simulink model "AllPurposeModel_TyreRelaxation"  (R2013b)
settings: Solver=ode45  StartTime=0.0  StopTime=16  FixedStep=0.001  MaxStep=0.01  RelTol=1e-3
StopFcn:
  | PlotPathAndForces(pos_irp3,delta_w4,F_z4,v_xv4,v_yv4,F_xv4,F_yv4, Par, -2);
  | TimePlots
undefined symbols (not defined in the file or in its folder): Par, sigbuilder_block
(part 1 of 2)
settings Model: DSRTSU_INTERNAL_RTI_VER=440  DSRTSU_INTERNAL_RTI_TYPE=rti1401  RTICANMMDATA=struct('GeneralSetupData',struct('modelroot','D:\Users\bengtja\Subversion_work\TM_VEAS_VD\CourseMaterial\MMF062_VehicleDynamics\Compendium\AllPurposeModel','generalsettings',struct('filesettings',struct('destfolder',struct('Name','RTICANMM_FILES','Check',1),'buildfolder',struct('Name','.','Check',1),'AbsDestfolder',struct('Name','D:\Users\bengtja\Subversion_work\TM_VEAS_VD\CourseMaterial\MMF062_VehicleDynamics\Compendium\AllPurposeModel\RTICANMM_FILES'),'AbsBuildfolder',struct('Name','D:\Users\bengtja\Subversion_work\TM_VEAS_VD\CourseMaterial\MMF062_VehicleDynamics\Compendium\AllPurposeModel'))),'options',struct('addpaths',1,'rmpaths',1,'addtrcexclusion',logical(1),'cannavigator',struct('checkmonitoring',0),'show_usrtrc',0,'use_usrtrc',0),'advanced',struct('options',[1 1 1 1 1 1 1 1 1 1 1 1 1 1 1 1 1 1 1 1 1 1 1 1 1 1 1 1 1 1 1 1 1 1 1 1 1 1 1 1 1 1 1 1 1 1 1 1 1 1 1 1 1 1 1 1 1 1 1 1 1 1 1 1 1 1 1 1 1 1 1 1 1 1 1 1 1 1 1 1 1 1 1 1 1 1 1 1 1 1 1 1 1 1 1 1 1 1 1 1]),'MPSetup',{{}},'modelname','AllPurposeModel','block','AllPurposeModel'))  DSRTSU_INTERNAL_RTIFPGA=30  BufferReuse=off  Creator=bengtja  LastModifiedBy=bengtja
settings OptimizationCC: BlockReduction=off  OptimizeBlockIOStorage=off  BufferReuse=off  ExpressionFolding=off  LocalBlockOutputs=off
settings DebuggingCC: ArtificialAlgebraicLoopMsg=none  StateNameClashWarn=warning
settings HardwareCC: ProdIntDivRoundTo=Zero  ProdEndianess=BigEndian  ProdHWDeviceType=Generic->Custom  TargetIntDivRoundTo=Zero  TargetEndianess=BigEndian  TargetHWDeviceType=Generic->Custom
settings RTWCC: SystemTargetFile=rti1401.tlc  MakeCommand=make_rti  TemplateMakefile=rti1401.tmf  Description=dSPACE DS1401 Hardware Platform  ProcessScript=rti1401_make_rtw_hook
settings STFCustomTargetCC: ParMdlRefBuildCompliant=on  GeneratePreprocessorConditionals=Disable all  MatFileLogging=on  SystemTargetFile=rti1401.tlc
settings GRTTargetCC: CompOptLevelCompliant=off  ConcurrentExecutionCompliant=off  CombineOutputUpdateFcns=off  GRTInterface=on  ExtModeMexFile=noextcomm

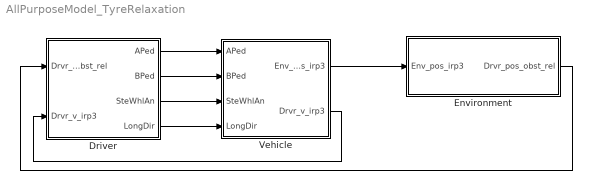
== system AllPurposeModel_TyreRelaxation ==
  Driver : Subsystem
  Environment : Subsystem
  Vehicle : Subsystem
  wires:
  Environment/1(Drvr_pos_obst_rel) -> Driver/1(Drvr_pos_obst_rel)
  Driver/1(APed) -> Vehicle/1(APed)
  Driver/2(BPed) -> Vehicle/2(BPed)
  Driver/3(SteWhlAn) -> Vehicle/3(SteWhlAn)
  Vehicle/2(Drvr_v_irp3) -> Driver/2(Drvr_v_irp3)
  Vehicle/1(Env_pos_irp3) -> Environment/1(Env_pos_irp3)
  Driver/4(LongDir) -> Vehicle/4(LongDir)

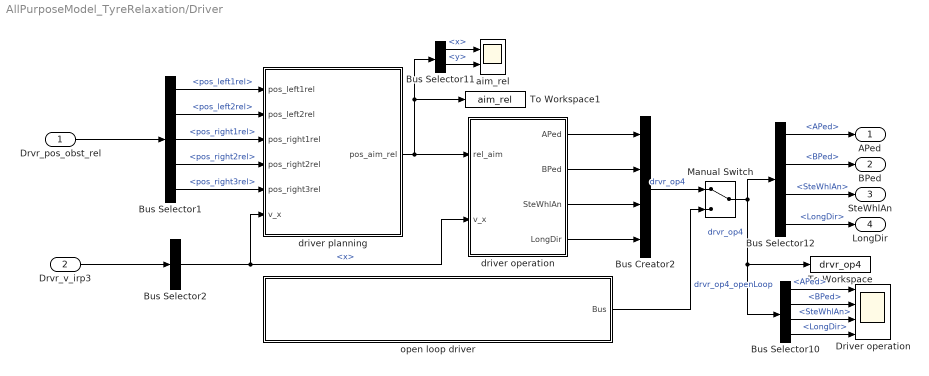
== system AllPurposeModel_TyreRelaxation/Driver ==
  Drvr_pos_obst_rel : Inport
  Drvr_v_irp3 : Inport  Port=2
  Bus Creator2 : BusCreator
  Bus Selector1 : BusSelector  OutputSignals=pos_left_rel.pos_left1rel,pos_left_rel.pos_left2rel,pos_right_rel.pos_right1rel,pos_right_rel.pos_right2rel,pos_right_rel.pos_right3rel
  Bus Selector10 : BusSelector  OutputSignals=APed,BPed,SteWhlAn,LongDir
  Bus Selector11 : BusSelector  OutputSignals=x,y
  Bus Selector12 : BusSelector  OutputSignals=APed,BPed,SteWhlAn,LongDir
  Bus Selector2 : BusSelector  OutputSignals=x
  Driver operation : Scope  NumInputPorts=4
      settings: YMin=-5.55112e-17~-1~-12.5~0.95  YMax=0.7~1~5~1.05
  Manual Switch : ManualSwitch
  To Workspace : ToWorkspace  VariableName=drvr_op4  SampleTime=-1  SaveFormat=Timeseries
  To Workspace1 : ToWorkspace  VariableName=aim_rel  SampleTime=-1  SaveFormat=Timeseries
  aim_rel : Scope  NumInputPorts=2
      settings: YMin=47.275~1.7525  YMax=47.65~1.785  SaveName=ScopeData5
  driver operation : MATLAB Function  TreatAsAtomicUnit=on
      settings: MinAlgLoopOccurrences=on
  driver planning : MATLAB Function  TreatAsAtomicUnit=on
      settings: MinAlgLoopOccurrences=on
  open loop driver : Subsystem  Tag=STV Subsys  LoadFcn=sigbuilder_block('load');  StartFcn=sigbuilder_block('start');  StopFcn=sigbuilder_block('stop');  ClipboardFcn=sigbuilder_block('clipboard');  mask(Sigbuilder block){}
      mask help: Simulink:masks:SigbuilderBlock_MD
      mask init:
      | if ~strcmp(get_param(bdroot(gcbh),'SimulationStatus'),'stopped') tuvar = sigbuilder_block('maskInit'); end
      settings: CopyFcn=sigbuilder_block('copy');  DeleteFcn=sigbuilder_block('delete');  ModelCloseFcn=sigbuilder_block('modelClose');  PreSaveFcn=sigbuilder_block('preSave');  PauseFcn=sigbuilder_block('pause');  ContinueFcn=sigbuilder_block('continue');  NameChangeFcn=sigbuilder_block('namechange');  OpenFcn=sigbuilder_block('open',[80.25 63.75 1019.25 535.5 ]);  CloseFcn=sigbuilder_block('close');
      mask Display: plot(0, 0, 100, 100,[2, 2, 32, 32, 2], [68, 8, 8, 68, 68],[32, 2], [38, 38], [32, 19, 2],[53, 60, 44], [32, 17, 17, 2],[16, 16, 31, 31]);txt = getActiveGroup(gcbh);text(2, 100, txt,'verticalAlignment', 'top');
  APed : Outport
  BPed : Outport  Port=2
  SteWhlAn : Outport  Port=3
  LongDir : Outport  Port=4
  wires:
  Drvr_pos_obst_rel/1 -> Bus Selector1/1
  Bus Selector1/3 -> driver planning/3(pos_right1rel)  "<pos_right1rel>"
  Bus Selector1/4 -> driver planning/4(pos_right2rel)  "<pos_right2rel>"
  driver operation/1(APed) -> Bus Creator2/1
  driver operation/2(BPed) -> Bus Creator2/2
  Bus Selector1/2 -> driver planning/2(pos_left2rel)  "<pos_left2rel>"
  Bus Selector1/1 -> driver planning/1(pos_left1rel)  "<pos_left1rel>"
  driver planning/1(pos_aim_rel) -> To Workspace1/1, Bus Selector11/1, driver operation/1(rel_aim)
  Bus Creator2/1 -> Manual Switch/1  "drvr_op4"
  Bus Selector10/2 -> Driver operation/2  "<BPed>"
  Bus Selector10/1 -> Driver operation/1  "<APed>"
  Bus Selector10/3 -> Driver operation/3  "<SteWhlAn>"
  Bus Selector11/2 -> aim_rel/2  "<y>"
  Bus Selector11/1 -> aim_rel/1  "<x>"
  Manual Switch/1 -> Bus Selector12/1, Bus Selector10/1, To Workspace/1  "drvr_op4"
  open loop driver/1(Bus) -> Manual Switch/2  "drvr_op4_openLoop"
  Bus Selector12/1 -> APed/1  "<APed>"
  Bus Selector12/2 -> BPed/1  "<BPed>"
  Bus Selector12/3 -> SteWhlAn/1  "<SteWhlAn>"
  driver operation/3(SteWhlAn) -> Bus Creator2/3
  Drvr_v_irp3/1 -> Bus Selector2/1
  Bus Selector2/1 -> driver operation/2(v_x), driver planning/6(v_x)  "<x>"
  driver operation/4(LongDir) -> Bus Creator2/4
  Bus Selector12/4 -> LongDir/1  "<LongDir>"
  Bus Selector10/4 -> Driver operation/4  "<LongDir>"
  Bus Selector1/5 -> driver planning/5(pos_right3rel)  "<pos_right3rel>"

== system AllPurposeModel_TyreRelaxation/Environment ==
  Env_pos_irp3 : Inport
  Bus Creator2 : BusCreator  Inputs=2
  Bus Creator3 : BusCreator  Inputs=3
  Bus Creator6 : BusCreator  Inputs=2
  Environment : MATLAB Function  TreatAsAtomicUnit=on
  Drvr_pos_obst_rel : Outport
  wires:
  Env_pos_irp3/1 -> Environment/1(pos_irp3)
  Environment/1(pos_left1rel) -> Bus Creator2/1
  Environment/2(pos_left2rel) -> Bus Creator2/2
  Environment/3(pos_right1rel) -> Bus Creator3/1
  Environment/4(pos_right2rel) -> Bus Creator3/2
  Bus Creator2/1 -> Bus Creator6/1  "pos_left_rel"
  Bus Creator3/1 -> Bus Creator6/2  "pos_right_rel"
  Bus Creator6/1 -> Drvr_pos_obst_rel/1  "Drvr_pos_obst_rel"
  Environment/5(pos_right3rel) -> Bus Creator3/3

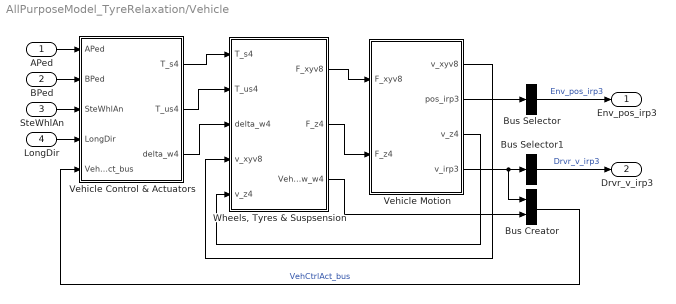
== system AllPurposeModel_TyreRelaxation/Vehicle ==
  APed : Inport
  BPed : Inport  Port=2
  SteWhlAn : Inport  Port=3
  LongDir : Inport  Port=4
  Bus Creator : BusCreator  Inputs=2
  Bus Selector : BusSelector  OutputSignals=x,y,rotz  OutputAsBus=on
  Bus Selector1 : BusSelector  OutputSignals=x,y,rotz  OutputAsBus=on
  Vehicle Control & Actuators : Subsystem
  Vehicle Motion : Subsystem
  "Wheels, Tyres & Suspsension" : Subsystem
  Env_pos_irp3 : Outport
  Drvr_v_irp3 : Outport  Port=2
  wires:
  Vehicle Motion/2(pos_irp3) -> Bus Selector/1
  BPed/1 -> Vehicle Control & Actuators/2(BPed)
  SteWhlAn/1 -> Vehicle Control & Actuators/3(SteWhlAn)
  APed/1 -> Vehicle Control & Actuators/1(APed)
  Vehicle Control & Actuators/2(T_us4) -> "Wheels, Tyres & Suspsension"/2(T_us4)
  Vehicle Control & Actuators/1(T_s4) -> "Wheels, Tyres & Suspsension"/1(T_s4)
  Vehicle Control & Actuators/3(delta_w4) -> "Wheels, Tyres & Suspsension"/3(delta_w4)
  "Wheels, Tyres & Suspsension"/1(F_xyv8) -> Vehicle Motion/1(F_xyv8)
  "Wheels, Tyres & Suspsension"/2(F_z4) -> Vehicle Motion/2(F_z4)
  Vehicle Motion/1(v_xyv8) -> "Wheels, Tyres & Suspsension"/4(v_xyv8)
  Vehicle Motion/3(v_z4) -> "Wheels, Tyres & Suspsension"/5(v_z4)
  Vehicle Motion/4(v_irp3) -> Bus Creator/1, Bus Selector1/1
  "Wheels, Tyres & Suspsension"/3(VehCtrlAct_w_w4) -> Bus Creator/2
  Bus Creator/1 -> Vehicle Control & Actuators/5(VehCtrlAct_bus)  "VehCtrlAct_bus"
  LongDir/1 -> Vehicle Control & Actuators/4(LongDir)
  Bus Selector/1 -> Env_pos_irp3/1  "Env_pos_irp3"
  Bus Selector1/1 -> Drvr_v_irp3/1  "Drvr_v_irp3"

== system AllPurposeModel_TyreRelaxation/Driver/open loop driver ==
  Bus Creator : BusCreator  Tag=Bus Creator
  FromWs : FromWorkspace  Tag=STV FromWs  VariableName=tuvar  SampleTime=0
      SigBuilderData=|
      | common.afterFinalStr = 'Extrapolate'
      | common.sampleTime = 0
      | dataSet.timeRange = [0 120]
      | dataSet.name = 'Group 1'
      | sbobj.Groups.Name = 'Group 1'
      | sbobj.Groups.Signals(1).Name = 'APed'
      | sbobj.Groups.Signals(1).XData = [0 2 10 10 30 30 40.1 40.1 70 120]
      | sbobj.Groups.Signals(1).YData = [0.01 0.01 0.49 0.5 0.5 1 1 0.5 0.49 0.49]
      | sbobj.Groups.Signals(2).Name = 'BPed'
      | sbobj.Groups.Signals(2).XData = [0 45 45 55 55 120]
      | sbobj.Groups.Signals(2).YData = [0 0 0.4 0.4 0 0]
      | sbobj.Groups.Signals(3).Name = 'SteWhlAn'
      | sbobj.Groups.Signals(3).XData = [0 60 80 90 100 120]
      | sbobj.Groups.Signals(3).YData = [0 0 0.2 0.2 0 0]
      | sbobj.Groups.Signals(4).Name = 'LongDir'
      | sbobj.Groups.Signals(4).XData = [0 120]
      | sbobj.Groups.Signals(4).YData = [1 1]
      | sbobj.Groups.TimeRange = [0 120]
  Subsystem : Subsystem
  Bus : Outport
  wires:
  FromWs/1 -> Subsystem/1(In1)
  Subsystem/1(APed) -> Bus Creator/1  "APed"
  Subsystem/2(BPed) -> Bus Creator/2  "BPed"
  Subsystem/3(SteWhlAn) -> Bus Creator/3  "SteWhlAn"
  Bus Creator/1 -> Bus/1
  Subsystem/4(LongDir) -> Bus Creator/4  "LongDir"

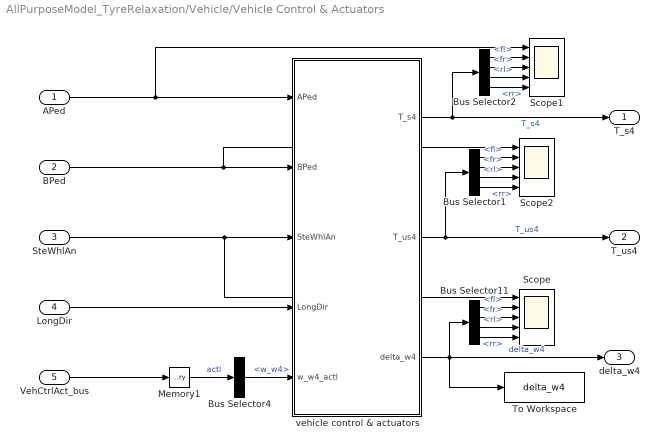
== system AllPurposeModel_TyreRelaxation/Vehicle/Vehicle Control & Actuators ==
  APed : Inport
  BPed : Inport  Port=2
  SteWhlAn : Inport  Port=3
  LongDir : Inport  Port=4
  VehCtrlAct_bus : Inport  Port=5
  Bus Selector1 : BusSelector  OutputSignals=fl,fr,rl,rr
  Bus Selector11 : BusSelector  OutputSignals=fl,fr,rl,rr
  Bus Selector2 : BusSelector  OutputSignals=fl,fr,rl,rr
  Bus Selector4 : BusSelector  OutputSignals=VehCtrlAct_w_w4.w_w4
  Memory1 : Memory  X0=Par.Init.v_x
  Scope : Scope  NumInputPorts=5
      settings: YMin=3562.5~-5~-5~-5~-5  YMax=3937.5~5~5~5~5  SaveName=ScopeData2
  Scope1 : Scope  NumInputPorts=5
      settings: YMin=5.55112e-17~0~0~-1~-1  YMax=1~700~700~1~1  SaveName=ScopeData10
  Scope2 : Scope  NumInputPorts=5
      settings: YMin=3562.5~-5~-5~-5~-5  YMax=3937.5~5~5~5~5  SaveName=ScopeData13
  To Workspace : ToWorkspace  VariableName=delta_w4  SampleTime=-1  SaveFormat=Timeseries
  vehicle control & actuators : MATLAB Function  TreatAsAtomicUnit=on
      settings: MinAlgLoopOccurrences=on
  T_s4 : Outport
  T_us4 : Outport  Port=2
  delta_w4 : Outport  Port=3
  wires:
  APed/1 -> vehicle control & actuators/1(APed), Scope1/1
  vehicle control & actuators/2(T_us4) -> Bus Selector1/1, T_us4/1  "T_us4"
  BPed/1 -> vehicle control & actuators/2(BPed), Scope2/1
  SteWhlAn/1 -> Scope/1, vehicle control & actuators/3(SteWhlAn)
  vehicle control & actuators/1(T_s4) -> T_s4/1, Bus Selector2/1  "T_s4"
  vehicle control & actuators/3(delta_w4) -> To Workspace/1, delta_w4/1, Bus Selector11/1  "delta_w4"
  Bus Selector2/3 -> Scope1/4  "<rl>"
  Bus Selector2/4 -> Scope1/5  "<rr>"
  Bus Selector2/1 -> Scope1/2  "<fl>"
  Bus Selector2/2 -> Scope1/3  "<fr>"
  Bus Selector11/4 -> Scope/5  "<rr>"
  Bus Selector11/3 -> Scope/4  "<rl>"
  Bus Selector11/2 -> Scope/3  "<fr>"
  Bus Selector11/1 -> Scope/2  "<fl>"
  Bus Selector1/3 -> Scope2/4  "<rl>"
  Bus Selector1/4 -> Scope2/5  "<rr>"
  Bus Selector1/1 -> Scope2/2  "<fl>"
  Bus Selector1/2 -> Scope2/3  "<fr>"
  VehCtrlAct_bus/1 -> Memory1/1
  Bus Selector4/1 -> vehicle control & actuators/5(w_w4_actl)  "<w_w4>"
  LongDir/1 -> vehicle control & actuators/4(LongDir)
  Memory1/1 -> Bus Selector4/1  "actl"

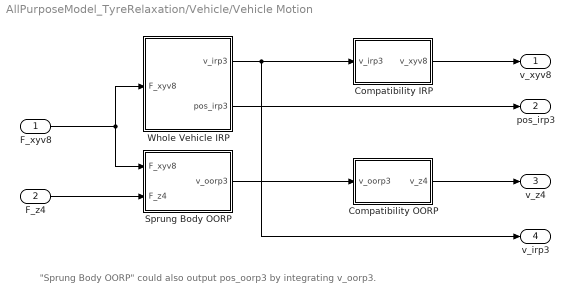
== system AllPurposeModel_TyreRelaxation/Vehicle/Vehicle Motion ==
  note: "Sprung Body OORP" could also output pos_oorp3 by integrating v_oorp3.
  F_xyv8 : Inport
  F_z4 : Inport  Port=2
  Compatibility IRP : Subsystem
  Compatibility OORP : Subsystem
  Sprung Body OORP : Subsystem
  Whole Vehicle IRP : Subsystem
  v_xyv8 : Outport
  pos_irp3 : Outport  Port=2
  v_z4 : Outport  Port=3
  v_irp3 : Outport  Port=4
  wires:
  F_xyv8/1 -> Whole Vehicle IRP/1(F_xyv8), Sprung Body OORP/1(F_xyv8)
  F_z4/1 -> Sprung Body OORP/2(F_z4)
  Sprung Body OORP/1(v_oorp3) -> Compatibility OORP/1(v_oorp3)
  Compatibility OORP/1(v_z4) -> v_z4/1
  Compatibility IRP/1(v_xyv8) -> v_xyv8/1
  Whole Vehicle IRP/1(v_irp3) -> v_irp3/1, Compatibility IRP/1(v_irp3)
  Whole Vehicle IRP/2(pos_irp3) -> pos_irp3/1

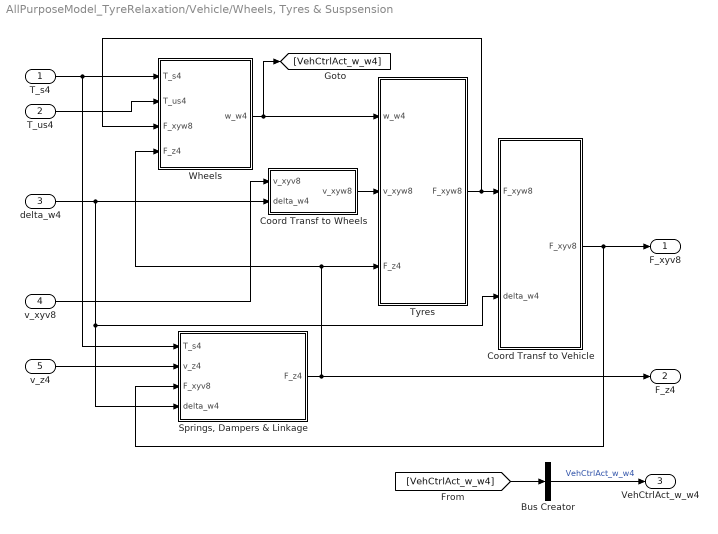
== system AllPurposeModel_TyreRelaxation/Vehicle/Wheels, Tyres & Suspsension ==
  T_s4 : Inport
  T_us4 : Inport  Port=2
  delta_w4 : Inport  Port=3
  v_xyv8 : Inport  Port=4
  v_z4 : Inport  Port=5
  Bus Creator : BusCreator  Inputs=1
  Coord Transf to Vehicle : Subsystem
      settings: MinAlgLoopOccurrences=on
  "Coord Transf to Wheels " : Subsystem
      settings: MinAlgLoopOccurrences=on
  "Springs, Dampers & Linkage" : Subsystem
      settings: MinAlgLoopOccurrences=on
  "Tyres " : Subsystem
      settings: MinAlgLoopOccurrences=on
  "Wheels " : Subsystem
      settings: MinAlgLoopOccurrences=on
  F_xyv8 : Outport
  F_z4 : Outport  Port=2
  VehCtrlAct_w_w4 : Outport  Port=3
  wires:
  "Tyres "/1(F_xyw8) -> "Wheels "/3(F_xyw8), Coord Transf to Vehicle/1(F_xyw8)
  "Coord Transf to Wheels "/1(v_xyw8) -> "Tyres "/2(v_xyw8)
  delta_w4/1 -> "Springs, Dampers & Linkage"/4(delta_w4), Coord Transf to Vehicle/2(delta_w4), "Coord Transf to Wheels "/2(delta_w4)
  "Wheels "/1(w_w4) -> [VehCtrlAct_w_w4], "Tyres "/1(w_w4)
  T_us4/1 -> "Wheels "/2(T_us4)
  v_xyv8/1 -> "Coord Transf to Wheels "/1(v_xyv8)
  Bus Creator/1 -> VehCtrlAct_w_w4/1  "VehCtrlAct_w_w4"
  [VehCtrlAct_w_w4] -> Bus Creator/1
  v_z4/1 -> "Springs, Dampers & Linkage"/2(v_z4)
  T_s4/1 -> "Springs, Dampers & Linkage"/1(T_s4), "Wheels "/1(T_s4)
  Coord Transf to Vehicle/1(F_xyv8) -> F_xyv8/1, "Springs, Dampers & Linkage"/3(F_xyv8)
  "Springs, Dampers & Linkage"/1(F_z4) -> F_z4/1, "Tyres "/3(F_z4), "Wheels "/4(F_z4)

== system AllPurposeModel_TyreRelaxation/Driver/open loop driver/Subsystem ==
  In1 : Inport
  Demux : Demux  Tag=STV Demux
  APed : Outport  Tag=STV Outport
  BPed : Outport  Tag=STV Outport  Port=2
  SteWhlAn : Outport  Tag=STV Outport  Port=3
  LongDir : Outport  Tag=STV Outport  Port=4
  wires:
  Demux/1 -> APed/1
  Demux/2 -> BPed/1
  Demux/3 -> SteWhlAn/1
  In1/1 -> Demux/1
  Demux/4 -> LongDir/1

== system AllPurposeModel_TyreRelaxation/Vehicle/Vehicle Motion/Compatibility IRP ==
  v_irp3 : Inport
  Bus Creator3 : BusCreator  Inputs=2
  Bus Selector1 : BusSelector  OutputSignals=fl,fr,rl,rr
  Bus Selector5 : BusSelector  OutputSignals=fl,fr,rl,rr
  Compatibility : MATLAB Function  TreatAsAtomicUnit=on
  Scope v_xv4 : Scope  NumInputPorts=4
      settings: YMin=0~0~63.3334~63.3334  YMax=80000~80000~70~70  SaveName=ScopeData24
  Scope v_yv4 : Scope  NumInputPorts=4
      settings: YMin=0~0~63.3334~63.3334  YMax=80000~80000~70~70  SaveName=ScopeData23
  To Workspace1 : ToWorkspace  VariableName=v_xv4  SampleTime=-1  SaveFormat=Timeseries
  To Workspace2 : ToWorkspace  VariableName=v_yv4  SampleTime=-1  SaveFormat=Timeseries
  v_xyv8 : Outport
  wires:
  v_irp3/1 -> Compatibility/1(v_irp3)
  Compatibility/1(v_xv4) -> Bus Creator3/1, To Workspace1/1, Bus Selector1/1  "v_xv4"
  Compatibility/2(v_yv4) -> Bus Creator3/2, To Workspace2/1, Bus Selector5/1  "v_yv4"
  Bus Creator3/1 -> v_xyv8/1  "v_xyv8"
  Bus Selector5/3 -> Scope v_yv4/3  "<rl>"
  Bus Selector5/2 -> Scope v_yv4/2  "<fr>"
  Bus Selector5/4 -> Scope v_yv4/4  "<rr>"
  Bus Selector1/3 -> Scope v_xv4/3  "<rl>"
  Bus Selector1/2 -> Scope v_xv4/2  "<fr>"
  Bus Selector1/4 -> Scope v_xv4/4  "<rr>"
  Bus Selector1/1 -> Scope v_xv4/1  "<fl>"
  Bus Selector5/1 -> Scope v_yv4/1  "<fl>"

== system AllPurposeModel_TyreRelaxation/Vehicle/Vehicle Motion/Compatibility OORP ==
  v_oorp3 : Inport
  Bus Selector1 : BusSelector  OutputSignals=fl,fr,rl,rr
  Compatibility Eq [1.11] : MATLAB Function  TreatAsAtomicUnit=on
  Scope v_z4 : Scope  NumInputPorts=4
      settings: YMin=-0.1~-0.025~-0.1~-0.025  YMax=0.03~0.125~0.03~0.125  SaveName=ScopeData25
  v_z4 : Outport
  wires:
  v_oorp3/1 -> Compatibility Eq [1.11]/1(v_oorp3)
  Compatibility Eq [1.11]/1(v_z4) -> v_z4/1, Bus Selector1/1
  Bus Selector1/1 -> Scope v_z4/1  "<fl>"
  Bus Selector1/3 -> Scope v_z4/3  "<rl>"
  Bus Selector1/2 -> Scope v_z4/2  "<fr>"
  Bus Selector1/4 -> Scope v_z4/4  "<rr>"

== system AllPurposeModel_TyreRelaxation/Vehicle/Vehicle Motion/Sprung Body OORP ==
  F_xyv8 : Inport
  F_z4 : Inport  Port=2
  Body OORP : MATLAB Function  TreatAsAtomicUnit=on
  Bus Selector1 : BusSelector  OutputSignals=F_xv4,F_yv4
  Bus Selector3 : BusSelector  OutputSignals=z,rotx,roty
  Bus Selector7 : BusSelector  OutputSignals=z,rotx,roty
  Integrator : Subsystem
  Scope v_irp3 : Scope  NumInputPorts=3
      settings: YMin=0~0~63.3334  YMax=80000~80000~70  SaveName=ScopeData9
  Scope2 : Scope  NumInputPorts=3
      settings: YMin=0~0~63.3334  YMax=80000~80000~70  SaveName=ScopeData14
  v_oorp3 : Outport
  wires:
  F_z4/1 -> Body OORP/3(F_z4)
  Bus Selector7/2 -> Scope v_irp3/2  "<rotx>"
  Bus Selector7/3 -> Scope v_irp3/3  "<roty>"
  Bus Selector7/1 -> Scope v_irp3/1  "<z>"
  Bus Selector3/2 -> Scope2/2  "<rotx>"
  Bus Selector3/3 -> Scope2/3  "<roty>"
  Bus Selector3/1 -> Scope2/1  "<z>"
  Body OORP/1(derv_oorp3) -> Bus Selector3/1, Integrator/1(derv_z)
  Integrator/1(v_oorp3) -> Bus Selector7/1, v_oorp3/1
  F_xyv8/1 -> Bus Selector1/1
  Bus Selector1/1 -> Body OORP/1(F_xv4)  "<F_xv4>"
  Bus Selector1/2 -> Body OORP/2(F_yv4)  "<F_yv4>"

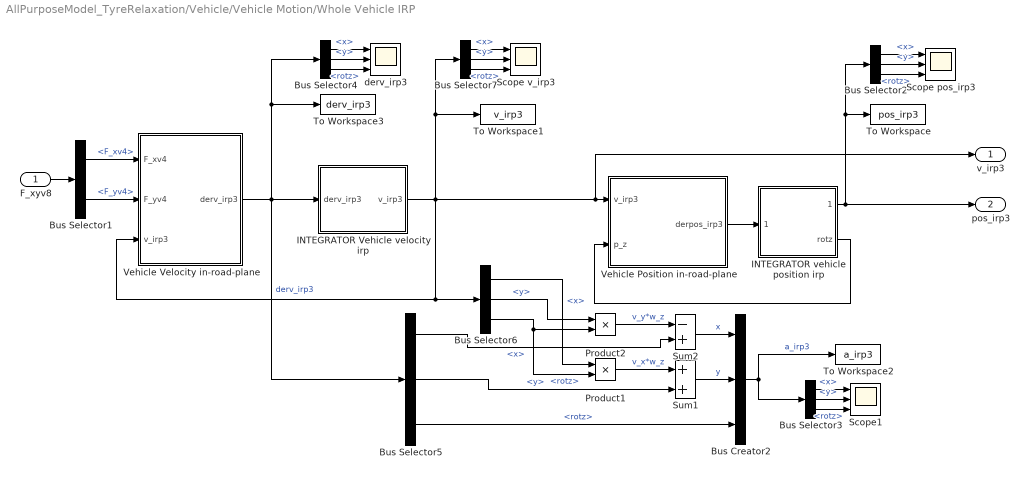
== system AllPurposeModel_TyreRelaxation/Vehicle/Vehicle Motion/Whole Vehicle IRP ==
  F_xyv8 : Inport
  Bus Creator2 : BusCreator  Inputs=3  OutDataTypeStr=Bus: irp_vec3
  Bus Selector1 : BusSelector  OutputSignals=F_xv4,F_yv4
  Bus Selector{2..7} (6 alike) : BusSelector  OutputSignals=x,y,rotz
  INTEGRATOR Vehicle velocity irp : Subsystem
  INTEGRATOR vehicle position irp : Subsystem
  Product1 : Product
  Product2 : Product
  Scope pos_irp3 : Scope  NumInputPorts=3
      settings: YMin=3~-1~2.5  YMax=11~1.5~20  SaveName=ScopeData6
  Scope v_irp3 : Scope  NumInputPorts=3
      settings: YMin=0~-1.5~-0.025  YMax=55~0.25~0.175
  Scope1 : Scope  NumInputPorts=3
      settings: YMin=-0.5~5.5~-0.03  YMax=0.25~9.25~0.08  SaveName=ScopeData21
  Sum1 : Sum
  Sum2 : Sum  Inputs=-+
  To Workspace : ToWorkspace  VariableName=pos_irp3  SampleTime=-1  SaveFormat=Timeseries
  To Workspace1 : ToWorkspace  VariableName=v_irp3  SampleTime=-1  SaveFormat=Timeseries
  To Workspace2 : ToWorkspace  VariableName=a_irp3  SampleTime=-1  SaveFormat=Timeseries
  To Workspace3 : ToWorkspace  VariableName=derv_irp3  SampleTime=-1  SaveFormat=Timeseries
  Vehicle Position in-road-plane : MATLAB Function  TreatAsAtomicUnit=on
  Vehicle Velocity in-road-plane : MATLAB Function  TreatAsAtomicUnit=on
  derv_irp3 : Scope  NumInputPorts=3
      settings: YMin=-0.2~0~0  YMax=-1.38778e-17~0.125~0.08  SaveName=ScopeData22
  v_irp3 : Outport
  pos_irp3 : Outport  Port=2
  wires:
  Bus Selector7/2 -> Scope v_irp3/2  "<y>"
  Bus Selector7/3 -> Scope v_irp3/3  "<rotz>"
  Bus Selector7/1 -> Scope v_irp3/1  "<x>"
  Bus Selector3/2 -> Scope1/2  "<y>"
  Bus Selector3/3 -> Scope1/3  "<rotz>"
  Bus Selector3/1 -> Scope1/1  "<x>"
  Bus Creator2/1 -> Bus Selector3/1, To Workspace2/1  "a_irp3"
  Bus Selector4/2 -> derv_irp3/2  "<y>"
  Bus Selector4/3 -> derv_irp3/3  "<rotz>"
  Bus Selector4/1 -> derv_irp3/1  "<x>"
  Product1/1 -> Sum1/1  "v_x*w_z"
  Sum1/1 -> Bus Creator2/2  "y"
  Sum2/1 -> Bus Creator2/1  "x"
  Product2/1 -> Sum2/1  "v_y*w_z"
  Vehicle Velocity in-road-plane/1(derv_irp3) -> Bus Selector4/1, To Workspace3/1, Bus Selector5/1, INTEGRATOR Vehicle velocity irp/1(derv_irp3)  "derv_irp3"
  INTEGRATOR Vehicle velocity irp/1(v_irp3) -> Vehicle Position in-road-plane/1(v_irp3), v_irp3/1, Bus Selector6/1, Vehicle Velocity in-road-plane/3(v_irp3), Bus Selector7/1, To Workspace1/1
  Bus Selector5/3 -> Bus Creator2/3  "<rotz>"
  Bus Selector5/2 -> Sum1/2  "<y>"
  Bus Selector5/1 -> Sum2/2  "<x>"
  Bus Selector6/2 -> Product2/1  "<y>"
  Bus Selector6/3 -> Product2/2, Product1/2  "<rotz>"
  Bus Selector6/1 -> Product1/1  "<x>"
  INTEGRATOR vehicle position irp/1(pos_irp3) -> Bus Selector2/1, To Workspace/1, pos_irp3/1
  Vehicle Position in-road-plane/1(derpos_irp3) -> INTEGRATOR vehicle position irp/1(derpos_irp3)
  INTEGRATOR vehicle position irp/2(rotz) -> Vehicle Position in-road-plane/2(p_z)
  F_xyv8/1 -> Bus Selector1/1
  Bus Selector1/1 -> Vehicle Velocity in-road-plane/1(F_xv4)  "<F_xv4>"
  Bus Selector1/2 -> Vehicle Velocity in-road-plane/2(F_yv4)  "<F_yv4>"
  Bus Selector2/2 -> Scope pos_irp3/2  "<y>"
  Bus Selector2/3 -> Scope pos_irp3/3  "<rotz>"
  Bus Selector2/1 -> Scope pos_irp3/1  "<x>"

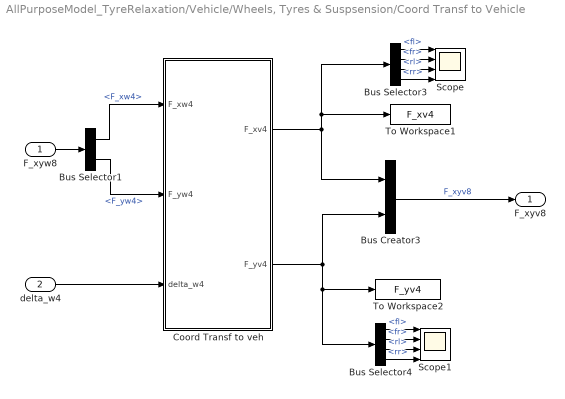
== system AllPurposeModel_TyreRelaxation/Vehicle/Wheels, Tyres & Suspsension/Coord Transf to Vehicle ==
  F_xyw8 : Inport
  delta_w4 : Inport  Port=2
  Bus Creator3 : BusCreator  Inputs=2
  Bus Selector1 : BusSelector  OutputSignals=F_xw4,F_yw4
  Bus Selector3 : BusSelector  OutputSignals=fl,fr,rl,rr
  Bus Selector4 : BusSelector  OutputSignals=fl,fr,rl,rr
  Coord Transf to veh : MATLAB Function  TreatAsAtomicUnit=on
      settings: MinAlgLoopOccurrences=on
  Scope : Scope  NumInputPorts=4
      settings: YMin=-0.5~-0.5~0~-4200  YMax=3.5~1.25~6000~-3400  SaveName=ScopeData3
  Scope1 : Scope  NumInputPorts=4
      settings: YMin=0~0~63.3334~63.3334  YMax=80000~80000~70~70  SaveName=ScopeData4
  To Workspace1 : ToWorkspace  VariableName=F_xv4  SampleTime=-1  SaveFormat=Timeseries
  To Workspace2 : ToWorkspace  VariableName=F_yv4  SampleTime=-1  SaveFormat=Timeseries
  F_xyv8 : Outport
  wires:
  delta_w4/1 -> Coord Transf to veh/3(delta_w4)
  Bus Selector3/1 -> Scope/1  "<fl>"
  Bus Selector3/3 -> Scope/3  "<rl>"
  Bus Selector3/2 -> Scope/2  "<fr>"
  Coord Transf to veh/1(F_xv4) -> Bus Creator3/1, To Workspace1/1, Bus Selector3/1
  Coord Transf to veh/2(F_yv4) -> Bus Creator3/2, To Workspace2/1, Bus Selector4/1
  Bus Selector3/4 -> Scope/4  "<rr>"
  Bus Selector4/3 -> Scope1/3  "<rl>"
  Bus Selector4/4 -> Scope1/4  "<rr>"
  Bus Selector4/2 -> Scope1/2  "<fr>"
  Bus Selector4/1 -> Scope1/1  "<fl>"
  F_xyw8/1 -> Bus Selector1/1
  Bus Creator3/1 -> F_xyv8/1  "F_xyv8"
  Bus Selector1/1 -> Coord Transf to veh/1(F_xw4)  "<F_xw4>"
  Bus Selector1/2 -> Coord Transf to veh/2(F_yw4)  "<F_yw4>"

== system AllPurposeModel_TyreRelaxation/Vehicle/Wheels, Tyres & Suspsension/Coord Transf to Wheels  ==
  v_xyv8 : Inport
  delta_w4 : Inport  Port=2
  Bus Creator4 : BusCreator  Inputs=2
  Bus Selector : BusSelector  OutputSignals=v_xv4,v_yv4
  Bus Selector4 : BusSelector  OutputSignals=fl,fr,rl,rr
  Bus Selector5 : BusSelector  OutputSignals=fl,fr,rl,rr
  Coord Transf to whl : MATLAB Function  TreatAsAtomicUnit=on
  Scope : Scope  NumInputPorts=4
      settings: YMin=0~0~63.3334~63.3334  YMax=80000~80000~70~70  SaveName=ScopeData7
  Scope1 : Scope  NumInputPorts=4
      settings: YMin=0~-50~0~-35  YMax=27.5~10~35~5  SaveName=ScopeData20
  v_xyw8 : Outport
  wires:
  v_xyv8/1 -> Bus Selector/1
  delta_w4/1 -> Coord Transf to whl/3(delta_w4)
  Bus Selector/1 -> Coord Transf to whl/1(v_xv4)  "<v_xv4>"
  Bus Selector/2 -> Coord Transf to whl/2(v_yv4)  "<v_yv4>"
  Bus Selector4/1 -> Scope/1  "<fl>"
  Bus Selector4/3 -> Scope/3  "<rl>"
  Bus Selector4/2 -> Scope/2  "<fr>"
  Bus Selector4/4 -> Scope/4  "<rr>"
  Bus Creator4/1 -> v_xyw8/1
  Coord Transf to whl/2(v_yw4) -> Bus Creator4/2, Bus Selector4/1
  Bus Selector5/1 -> Scope1/1  "<fl>"
  Bus Selector5/3 -> Scope1/3  "<rl>"
  Bus Selector5/2 -> Scope1/2  "<fr>"
  Bus Selector5/4 -> Scope1/4  "<rr>"
  Coord Transf to whl/1(v_xw4) -> Bus Creator4/1, Bus Selector5/1

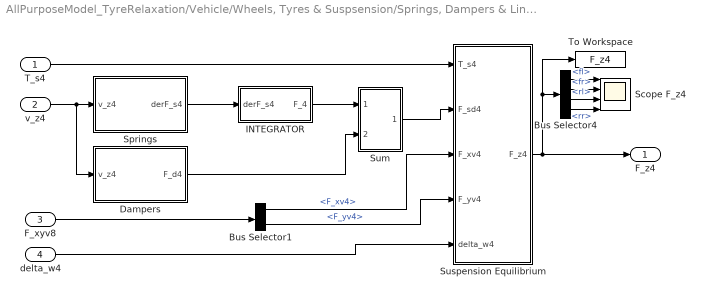
== system AllPurposeModel_TyreRelaxation/Vehicle/Wheels, Tyres & Suspsension/Springs, Dampers & Linkage ==
  T_s4 : Inport
  v_z4 : Inport  Port=2
  F_xyv8 : Inport  Port=3
  delta_w4 : Inport  Port=4
  Bus Selector1 : BusSelector  OutputSignals=F_xv4,F_yv4
  Bus Selector4 : BusSelector  OutputSignals=fl,fr,rl,rr
  Dampers : MATLAB Function  TreatAsAtomicUnit=on
      settings: MinAlgLoopOccurrences=on
  INTEGRATOR : Subsystem
  Scope F_z4 : Scope  NumInputPorts=4
      settings: YMin=4170~4165~4120~4120  YMax=4225~4220~4170~4165  SaveName=ScopeData17
  Springs : MATLAB Function  TreatAsAtomicUnit=on
      settings: MinAlgLoopOccurrences=on
  Sum : Subsystem
      settings: MinAlgLoopOccurrences=on
  Suspension Equilibrium : MATLAB Function  TreatAsAtomicUnit=on
      settings: MinAlgLoopOccurrences=on
  To Workspace : ToWorkspace  VariableName=F_z4  SampleTime=-1  SaveFormat=Timeseries
  F_z4 : Outport
  wires:
  T_s4/1 -> Suspension Equilibrium/1(T_s4)
  Bus Selector4/1 -> Scope F_z4/1  "<fl>"
  Bus Selector4/3 -> Scope F_z4/3  "<rl>"
  Bus Selector4/2 -> Scope F_z4/2  "<fr>"
  Bus Selector4/4 -> Scope F_z4/4  "<rr>"
  v_z4/1 -> Dampers/1(v_z4), Springs/1(v_z4)
  Springs/1(derF_s4) -> INTEGRATOR/1(derF_s4)
  INTEGRATOR/1(F_4) -> Sum/1(F_s4)
  Sum/1(F_sd4) -> Suspension Equilibrium/2(F_sd4)
  Suspension Equilibrium/1(F_z4) -> Bus Selector4/1, To Workspace/1, F_z4/1
  Bus Selector1/1 -> Suspension Equilibrium/3(F_xv4)  "<F_xv4>"
  Bus Selector1/2 -> Suspension Equilibrium/4(F_yv4)  "<F_yv4>"
  Dampers/1(F_d4) -> Sum/2(F_d4)
  F_xyv8/1 -> Bus Selector1/1
  delta_w4/1 -> Suspension Equilibrium/5(delta_w4)

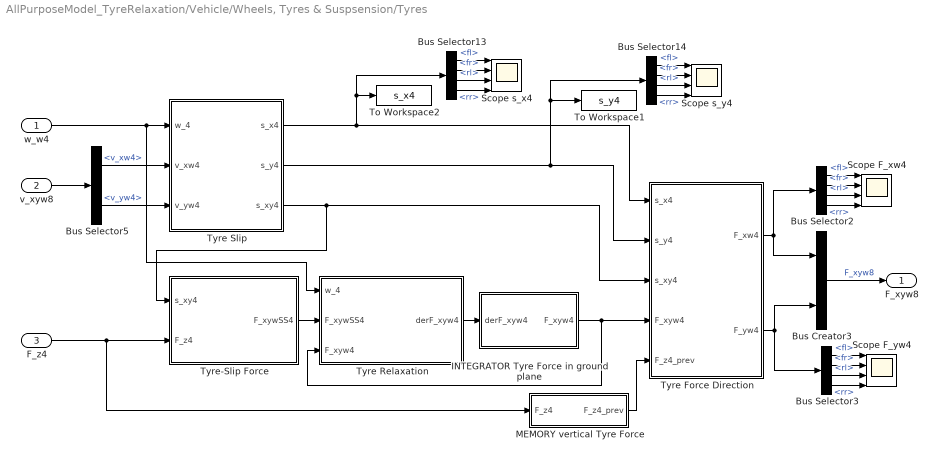
== system AllPurposeModel_TyreRelaxation/Vehicle/Wheels, Tyres & Suspsension/Tyres  ==
  w_w4 : Inport
  v_xyw8 : Inport  Port=2
  F_z4 : Inport  Port=3
  " MEMORY vertical Tyre Force" : Subsystem
      settings: MinAlgLoopOccurrences=on
  Bus Creator3 : BusCreator  Inputs=2
  Bus Selector{2..3,13..14} (4 alike) : BusSelector  OutputSignals=fl,fr,rl,rr
  Bus Selector5 : BusSelector  OutputSignals=v_xw4,v_yw4
  INTEGRATOR Tyre Force in ground plane : Subsystem
      settings: MinAlgLoopOccurrences=on
  Scope F_xw4 : Scope  NumInputPorts=4
      settings: YMin=0~-100~-0.05~-12.5  YMax=700~700~0.2~2.5  SaveName=ScopeData18
  Scope F_yw4 : Scope  NumInputPorts=4
      settings: YMin=-1000~0~-3500~-60000  YMax=5000~60000~1000~0  SaveName=ScopeData19
  Scope s_x4 : Scope  NumInputPorts=4
      settings: YMin=-0.0025~-0.0025~-0.00025~-0.0002  YMax=0.025~0.025~5e-05~0  SaveName=ScopeData11
  Scope s_y4 : Scope  NumInputPorts=4
      settings: YMin=-0.007~-0.008~-0.006~-0.006  YMax=0.001~0~0~0  SaveName=ScopeData12
  To Workspace1 : ToWorkspace  VariableName=s_y4  SampleTime=-1  SaveFormat=Timeseries
  To Workspace2 : ToWorkspace  VariableName=s_x4  SampleTime=-1  SaveFormat=Timeseries
  Tyre Force Direction : MATLAB Function
  Tyre Relaxation : MATLAB Function  TreatAsAtomicUnit=on
      settings: MinAlgLoopOccurrences=on
  Tyre Slip : MATLAB Function  TreatAsAtomicUnit=on
      settings: MinAlgLoopOccurrences=on
  Tyre-Slip Force : MATLAB Function  TreatAsAtomicUnit=on
      settings: MinAlgLoopOccurrences=on
  F_xyw8 : Outport
  wires:
  w_w4/1 -> Tyre Relaxation/1(w_4), Tyre Slip/1(w_4)
  v_xyw8/1 -> Bus Selector5/1
  Tyre Slip/1(s_x4) -> Tyre Force Direction/1(s_x4), To Workspace2/1, Bus Selector13/1
  Tyre Slip/2(s_y4) -> Tyre Force Direction/2(s_y4), To Workspace1/1, Bus Selector14/1
  Bus Selector13/3 -> Scope s_x4/3  "<rl>"
  Bus Selector13/4 -> Scope s_x4/4  "<rr>"
  Bus Selector13/2 -> Scope s_x4/2  "<fr>"
  Bus Selector13/1 -> Scope s_x4/1  "<fl>"
  Bus Selector14/3 -> Scope s_y4/3  "<rl>"
  Bus Selector14/4 -> Scope s_y4/4  "<rr>"
  Bus Selector14/2 -> Scope s_y4/2  "<fr>"
  Bus Selector14/1 -> Scope s_y4/1  "<fl>"
  Bus Selector2/3 -> Scope F_xw4/3  "<rl>"
  Bus Selector2/4 -> Scope F_xw4/4  "<rr>"
  Bus Selector2/2 -> Scope F_xw4/2  "<fr>"
  Bus Selector2/1 -> Scope F_xw4/1  "<fl>"
  Bus Selector3/3 -> Scope F_yw4/3  "<rl>"
  Bus Selector3/4 -> Scope F_yw4/4  "<rr>"
  Bus Selector3/2 -> Scope F_yw4/2  "<fr>"
  Bus Selector3/1 -> Scope F_yw4/1  "<fl>"
  Bus Creator3/1 -> F_xyw8/1  "F_xyw8"
  Tyre Relaxation/1(derF_xyw4) -> INTEGRATOR Tyre Force in ground plane/1(derF_xyw4)
  INTEGRATOR Tyre Force in ground plane/1(F_xyw4) -> Tyre Force Direction/4(F_xyw4), Tyre Relaxation/3(F_xyw4)
  Tyre Force Direction/1(F_xw4) -> Bus Creator3/1, Bus Selector2/1
  Tyre Force Direction/2(F_yw4) -> Bus Creator3/2, Bus Selector3/1
  Tyre Slip/3(s_xy4) -> Tyre Force Direction/3(s_xy4), Tyre-Slip Force/1(s_xy4)
  Bus Selector5/1 -> Tyre Slip/2(v_xw4)  "<v_xw4>"
  Bus Selector5/2 -> Tyre Slip/3(v_yw4)  "<v_yw4>"
  Tyre-Slip Force/1(F_xywSS4) -> Tyre Relaxation/2(F_xywSS4)
  F_z4/1 -> " MEMORY vertical Tyre Force"/1(F_z4), Tyre-Slip Force/2(F_z4)
  " MEMORY vertical Tyre Force"/1(F_z4_prev) -> Tyre Force Direction/5(F_z4_prev)

== system AllPurposeModel_TyreRelaxation/Vehicle/Wheels, Tyres & Suspsension/Wheels  ==
  T_s4 : Inport
  T_us4 : Inport  Port=2
  F_xyw8 : Inport  Port=3
  F_z4 : Inport  Port=4
  Bus Selector1 : BusSelector  OutputSignals=F_xw4,F_yw4
  Bus Selector6 : BusSelector  OutputSignals=fl,fr,rl,rr
  INTEGRATOR : Subsystem
  Scope w_w4 : Scope  NumInputPorts=4
      settings: YMin=-7500~-10000~-50000~-50000  YMax=32500~30000~5000~5000  SaveName=ScopeData15
  "Wheels " : MATLAB Function  TreatAsAtomicUnit=on
  w_w4 : Outport
  wires:
  T_us4/1 -> "Wheels "/2(T_us4)
  T_s4/1 -> "Wheels "/1(T_s4)
  Bus Selector6/4 -> Scope w_w4/4  "<rr>"
  Bus Selector6/3 -> Scope w_w4/3  "<rl>"
  Bus Selector6/1 -> Scope w_w4/1  "<fl>"
  Bus Selector6/2 -> Scope w_w4/2  "<fr>"
  "Wheels "/1(derw_w4) -> INTEGRATOR/1(derw_w4)
  F_z4/1 -> "Wheels "/5(F_z4)
  F_xyw8/1 -> Bus Selector1/1
  Bus Selector1/2 -> "Wheels "/4(F_yv4)  "<F_yw4>"
  Bus Selector1/1 -> "Wheels "/3(F_xv4)  "<F_xw4>"
  INTEGRATOR/1(w_w4) -> w_w4/1, "Wheels "/6(w_w4), Bus Selector6/1

== system AllPurposeModel_TyreRelaxation/Vehicle/Vehicle Motion/Sprung Body OORP/Integrator ==
  derv_z : Inport
  Bus Creator : BusCreator  Inputs=3  OutDataTypeStr=Bus: oorp_vec3
  Bus Selector4 : BusSelector  OutputSignals=z,rotx,roty
  Integ Heave : Integrator
  Integ Pitch : Integrator
  Integ Roll : Integrator
  v_oorp3 : Outport
  wires:
  Integ Pitch/1 -> Bus Creator/3  "roty"
  Integ Heave/1 -> Bus Creator/1  "z"
  Integ Roll/1 -> Bus Creator/2  "rotx"
  Bus Creator/1 -> v_oorp3/1  "v_oorp3"
  derv_z/1 -> Bus Selector4/1
  Bus Selector4/1 -> Integ Heave/1  "<z>"
  Bus Selector4/2 -> Integ Roll/1  "<rotx>"
  Bus Selector4/3 -> Integ Pitch/1  "<roty>"

== system AllPurposeModel_TyreRelaxation/Vehicle/Vehicle Motion/Whole Vehicle IRP/INTEGRATOR Vehicle velocity irp ==
  derv_irp3 : Inport
  Bus Creator : BusCreator  Inputs=3  OutDataTypeStr=Bus: irp_vec3
  Bus Selector : BusSelector  OutputSignals=x,y,rotz
  Integ Lat : Integrator
  Integ Long : Integrator  InitialCondition=Par.Init.v_x
  Integ Yaw : Integrator
  v_irp3 : Outport
  wires:
  Bus Creator/1 -> v_irp3/1  "v_irp3"
  Bus Selector/3 -> Integ Yaw/1  "<rotz>"
  Bus Selector/1 -> Integ Long/1  "<x>"
  Integ Long/1 -> Bus Creator/1  "x"
  derv_irp3/1 -> Bus Selector/1
  Bus Selector/2 -> Integ Lat/1  "<y>"
  Integ Lat/1 -> Bus Creator/2  "y"
  Integ Yaw/1 -> Bus Creator/3  "rotz"

== system AllPurposeModel_TyreRelaxation/Vehicle/Vehicle Motion/Whole Vehicle IRP/INTEGRATOR vehicle position irp ==
  derpos_irp3 : Inport
  Bus Creator3 : BusCreator  Inputs=3  OutDataTypeStr=Bus: irp_vec3
  Bus Selector2 : BusSelector  OutputSignals=x,y,rotz
  Integ p_z : Integrator
  Integ x : Integrator
  Integ y : Integrator
  pos_irp3 : Outport
  rotz : Outport  Port=2
  wires:
  derpos_irp3/1 -> Bus Selector2/1
  Integ y/1 -> Bus Creator3/2  "y"
  Integ p_z/1 -> rotz/1, Bus Creator3/3  "rotz"
  Integ x/1 -> Bus Creator3/1  "x"
  Bus Creator3/1 -> pos_irp3/1  "pos_irp3"
  Bus Selector2/3 -> Integ p_z/1  "<rotz>"
  Bus Selector2/1 -> Integ x/1  "<x>"
  Bus Selector2/2 -> Integ y/1  "<y>"

== system AllPurposeModel_TyreRelaxation/Vehicle/Wheels, Tyres & Suspsension/Springs, Dampers & Linkage/INTEGRATOR ==
  derF_s4 : Inport
  Bus Creator3 : BusCreator
  Bus Selector7 : BusSelector  OutputSignals=fl,fr,rl,rr
  Integrator1 : Integrator  InitialCondition=Par.Init.F_fz/2
  Integrator2 : Integrator  InitialCondition=Par.Init.F_fz/2
  Integrator3 : Integrator  InitialCondition=Par.Init.F_rz/2
  Integrator4 : Integrator  InitialCondition=Par.Init.F_rz/2
  F_4 : Outport
  wires:
  Integrator1/1 -> Bus Creator3/1  "fl"
  Integrator3/1 -> Bus Creator3/3  "rl"
  Integrator4/1 -> Bus Creator3/4  "rr"
  Integrator2/1 -> Bus Creator3/2  "fr"
  derF_s4/1 -> Bus Selector7/1
  Bus Selector7/1 -> Integrator1/1  "<fl>"
  Bus Creator3/1 -> F_4/1  "F_s4"
  Bus Selector7/2 -> Integrator2/1  "<fr>"
  Bus Selector7/4 -> Integrator4/1  "<rr>"
  Bus Selector7/3 -> Integrator3/1  "<rl>"

== system AllPurposeModel_TyreRelaxation/Vehicle/Wheels, Tyres & Suspsension/Springs, Dampers & Linkage/Sum ==
  F_s4 : Inport
  F_d4 : Inport  Port=2
  Bus Creator4 : BusCreator
  Bus Selector7 : BusSelector  OutputSignals=fl,fr,rl,rr
  Bus Selector8 : BusSelector  OutputSignals=fl,fr,rl,rr
  Sum{1..4} (4 alike) : Sum
  F_sd4 : Outport
  wires:
  Sum3/1 -> Bus Creator4/3  "rl"
  Sum4/1 -> Bus Creator4/4  "rr"
  Sum1/1 -> Bus Creator4/1  "fl"
  Sum2/1 -> Bus Creator4/2  "fr"
  Bus Selector8/1 -> Sum1/2  "<fl>"
  F_d4/1 -> Bus Selector8/1
  F_s4/1 -> Bus Selector7/1
  Bus Selector7/3 -> Sum3/1  "<rl>"
  Bus Selector7/4 -> Sum4/1  "<rr>"
  Bus Selector7/2 -> Sum2/1  "<fr>"
  Bus Selector7/1 -> Sum1/1  "<fl>"
  Bus Creator4/1 -> F_sd4/1  "F_sd4"
  Bus Selector8/4 -> Sum4/2  "<rr>"
  Bus Selector8/3 -> Sum3/2  "<rl>"
  Bus Selector8/2 -> Sum2/2  "<fr>"

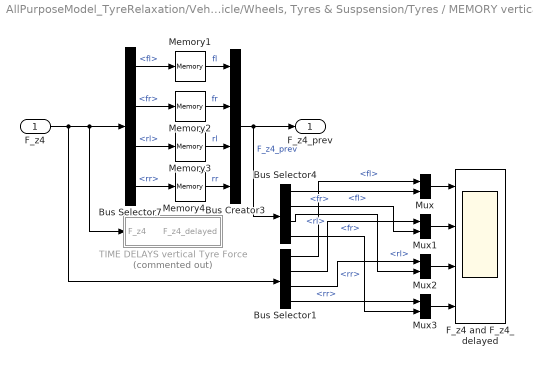
== system AllPurposeModel_TyreRelaxation/Vehicle/Wheels, Tyres & Suspsension/Tyres / MEMORY vertical Tyre Force ==
  F_z4 : Inport
  Bus Creator3 : BusCreator
  Bus Selector1 : BusSelector  OutputSignals=fl,fr,rl,rr
  Bus Selector4 : BusSelector  OutputSignals=fl,fr,rl,rr
  Bus Selector7 : BusSelector  OutputSignals=fl,fr,rl,rr
  F_z4 and F_z4_delayed : Scope  NumInputPorts=4
      settings: YMin=2000~1000~1000~1000  YMax=9000~8000~6000~5500  SaveName=ScopeData16
  Memory{1..4} (4 alike) : Memory
  Mux{,1..3} (4 alike) : Mux  Inputs=2
  TIME DELAYS vertical Tyre Force : Subsystem  Commented=on
      settings: MinAlgLoopOccurrences=on
  F_z4_prev : Outport
  wires:
  Memory1/1 -> Bus Creator3/1  "fl"
  Memory3/1 -> Bus Creator3/3  "rl"
  Memory4/1 -> Bus Creator3/4  "rr"
  Memory2/1 -> Bus Creator3/2  "fr"
  F_z4/1 -> Bus Selector1/1, TIME DELAYS vertical Tyre Force/1(F_z4), Bus Selector7/1
  Bus Selector7/1 -> Memory1/1  "<fl>"
  Bus Creator3/1 -> Bus Selector4/1, F_z4_prev/1  "F_z4_prev"
  Bus Selector7/2 -> Memory2/1  "<fr>"
  Bus Selector7/4 -> Memory4/1  "<rr>"
  Bus Selector7/3 -> Memory3/1  "<rl>"
  Bus Selector4/1 -> Mux/2  "<fl>"
  Mux/1 -> F_z4 and F_z4_delayed/1
  Bus Selector1/1 -> Mux/1  "<fl>"
  Mux1/1 -> F_z4 and F_z4_delayed/2
  Mux2/1 -> F_z4 and F_z4_delayed/3
  Mux3/1 -> F_z4 and F_z4_delayed/4
  Bus Selector1/2 -> Mux1/1  "<fr>"
  Bus Selector1/3 -> Mux2/1  "<rl>"
  Bus Selector1/4 -> Mux3/1  "<rr>"
  Bus Selector4/3 -> Mux2/2  "<rl>"
  Bus Selector4/4 -> Mux3/2  "<rr>"
  Bus Selector4/2 -> Mux1/2  "<fr>"

== system AllPurposeModel_TyreRelaxation/Vehicle/Wheels, Tyres & Suspsension/Tyres /INTEGRATOR Tyre Force in ground plane ==
  derF_xyw4 : Inport
  Bus Creator3 : BusCreator
  Bus Selector7 : BusSelector  OutputSignals=fl,fr,rl,rr
  Integrator{1..4} (4 alike) : Integrator
  F_xyw4 : Outport
  wires:
  Integrator1/1 -> Bus Creator3/1  "fl"
  Integrator3/1 -> Bus Creator3/3  "rl"
  Integrator4/1 -> Bus Creator3/4  "rr"
  Integrator2/1 -> Bus Creator3/2  "fr"
  derF_xyw4/1 -> Bus Selector7/1
  Bus Selector7/1 -> Integrator1/1  "<fl>"
  Bus Creator3/1 -> F_xyw4/1  "F_xvw4"
  Bus Selector7/2 -> Integrator2/1  "<fr>"
  Bus Selector7/4 -> Integrator4/1  "<rr>"
  Bus Selector7/3 -> Integrator3/1  "<rl>"

== system AllPurposeModel_TyreRelaxation/Vehicle/Wheels, Tyres & Suspsension/Wheels /INTEGRATOR ==
  derw_w4 : Inport
  Bus Creator1 : BusCreator
  Bus Selector1 : BusSelector  OutputSignals=fl,fr,rl,rr
  Integ Whl{1..4} (4 alike) : Integrator  InitialCondition=Par.Init.v_x/Par.Veh.Rw
  w_w4 : Outport
  wires:
  Integ Whl1/1 -> Bus Creator1/1  "fl"
  Bus Creator1/1 -> w_w4/1  "w_w4"
  Integ Whl4/1 -> Bus Creator1/4  "rr"
  Integ Whl3/1 -> Bus Creator1/3  "rl"
  Integ Whl2/1 -> Bus Creator1/2  "fr"
  Bus Selector1/4 -> Integ Whl4/1  "<rr>"
  Bus Selector1/2 -> Integ Whl2/1  "<fr>"
  Bus Selector1/1 -> Integ Whl1/1  "<fl>"
  Bus Selector1/3 -> Integ Whl3/1  "<rl>"
  derw_w4/1 -> Bus Selector1/1

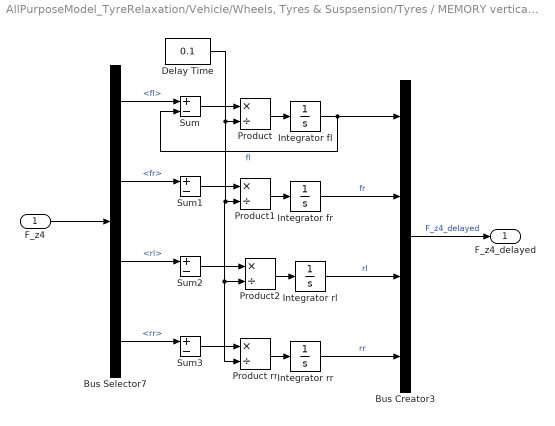
== system AllPurposeModel_TyreRelaxation/Vehicle/Wheels, Tyres & Suspsension/Tyres / MEMORY vertical Tyre Force/TIME DELAYS vertical Tyre Force ==
  F_z4 : Inport
  Bus Creator3 : BusCreator
  Bus Selector7 : BusSelector  OutputSignals=fl,fr,rl,rr
  Delay Time : Constant  Value=0.1
  Integrator fl : Integrator
  Integrator fr : Integrator
  Integrator rl : Integrator
  Integrator rr : Integrator
  Product : Product  Inputs=*/
  Product rr : Product  Inputs=*/
  Product1 : Product  Inputs=*/
  Product2 : Product  Inputs=*/
  Sum{,1..3} (4 alike) : Sum  Inputs=+-
  F_z4_delayed : Outport
  wires:
  Integrator fl/1 -> Bus Creator3/1, Sum/2  "fl"
  Integrator rl/1 -> Bus Creator3/3  "rl"
  Integrator rr/1 -> Bus Creator3/4  "rr"
  Integrator fr/1 -> Bus Creator3/2  "fr"
  F_z4/1 -> Bus Selector7/1
  Bus Selector7/1 -> Sum/1  "<fl>"
  Bus Creator3/1 -> F_z4_delayed/1  "F_z4_delayed"
  Bus Selector7/2 -> Sum1/1  "<fr>"
  Bus Selector7/4 -> Sum3/1  "<rr>"
  Bus Selector7/3 -> Sum2/1  "<rl>"
  Sum/1 -> Product/1
  Product/1 -> Integrator fl/1
  Delay Time/1 -> Product2/2, Product rr/2, Product1/2, Product/2
  Sum1/1 -> Product1/1
  Product1/1 -> Integrator fr/1
  Sum2/1 -> Product2/1
  Product2/1 -> Integrator rl/1
  Sum3/1 -> Product rr/1
  Product rr/1 -> Integrator rr/1

== matlab function AllPurposeModel_TyreRelaxation/Driver/driver operation ==
  data: APed output; BPed output; SteWhlAn output; rel_aim input; v_x input; Par parameter; LongDir output
function [APed, BPed, SteWhlAn, LongDir] = Driver(rel_aim, v_x, Par)
%#codegen

%%% Lane change between cones. Assumes SteWhlAn as state variable outside Matlab script block
Ped=1*(Par.Drvr.v_set-v_x);
APed=+min([+max([Ped,0]), +1]);
BPed=-max([+min([Ped,0]), -1]);

L=Par.Veh.L;
W=Par.Veh.TrackWidth;
lr=Par.Veh.lr;

arg_arcsin=(2*L*rel_aim.y)/((lr - rel_aim.x)^2 + rel_aim.y^2);
if abs(arg_arcsin)<=1
    d1 = asin(arg_arcsin);
    d2 = pi - d1;
    if abs(d1)<abs(d2), d=d1; else, d=d2; end
    SteWhlAn=Par.Veh.SteRatio*sign(d)*min(abs(d), pi/4); %steering lock at 45 deg = pi/4 rad
else
    SteWhlAn=0; %give up steering
end

LongDir=1; %LongDir is -1 or +1

== matlab function AllPurposeModel_TyreRelaxation/Driver/driver planning ==
  data: pos_left1rel input Bus: obst_vec2; pos_left2rel input Bus: obst_vec2; pos_right1rel input Bus: obst_vec2; pos_right2rel input Bus: obst_vec2; pos_right3rel input; v_x input; pos_aim_rel output Bus: obst_vec2; Par parameter
function pos_aim_rel = Driver(pos_left1rel, pos_left2rel, pos_right1rel, pos_right2rel, pos_right3rel, v_x, Par)
%#codegen

dist_left1rel=sqrt(pos_left1rel.x^2+pos_left1rel.y^2);
dist_left2rel=sqrt(pos_left2rel.x^2+pos_left2rel.y^2);
dist_right1rel=sqrt(pos_right1rel.x^2+pos_right1rel.y^2);
dist_right2rel=sqrt(pos_right2rel.x^2+pos_right2rel.y^2);
dist_right3rel=sqrt(pos_right3rel.x^2+pos_right3rel.y^2);

dist_select_rel=inf;
pos_aim_rel.x=100; %look ahead...
pos_aim_rel.y=0; %drive straigth...

if pos_left1rel.x>Par.Veh.lf & dist_left1rel<dist_select_rel
    pos_aim_rel.x=pos_left1rel.x;
    pos_aim_rel.y=pos_left1rel.y;
    dist_select_rel=dist_left1rel;
end

if pos_left2rel.x>Par.Veh.lf & dist_left2rel<dist_select_rel
    pos_aim_rel.x=pos_left2rel.x;
    pos_aim_rel.y=pos_left2rel.y;
    dist_select_rel=dist_left2rel;
end

if pos_right1rel.x>Par.Veh.lf & dist_right1rel<dist_select_rel
    pos_aim_rel.x=pos_right1rel.x;
    pos_aim_rel.y=pos_right1rel.y;
    dist_select_rel=dist_right1rel;
end

if pos_right2rel.x>Par.Veh.lf & dist_right2rel<dist_select_rel
    pos_aim_rel.x=pos_right2rel.x;
    pos_aim_rel.y=pos_right2rel.y;
    dist_select_rel=dist_right2rel;
end

if pos_right3rel.x>Par.Veh.lf & dist_right3rel<dist_select_rel
    pos_aim_rel.x=pos_right3rel.x;
    pos_aim_rel.y=pos_right3rel.y;
    dist_select_rel=dist_right3rel;
end

== matlab function AllPurposeModel_TyreRelaxation/Vehicle/Wheels, Tyres & Suspsension/Tyres /Tyre Slip ==
  data: w_4 input Bus: whl_vec4; v_xw4 input Bus: whl_vec4; v_yw4 input Bus: whl_vec4; s_x4 output Bus: whl_vec4; s_y4 output Bus: whl_vec4; Par parameter; s_xy4 output Bus: whl_vec4
function [s_x4, s_y4, s_xy4] = TyreModel(w_4, v_xw4, v_yw4, Par)
%#codegen

Rw=Par.Veh.Rw;

s_x4.fl=(Rw*w_4.fl-v_xw4.fl)/(abs(Rw*w_4.fl+v_xw4.fl)/2);
s_x4.fr=(Rw*w_4.fr-v_xw4.fr)/(abs(Rw*w_4.fr+v_xw4.fr)/2);
s_x4.rl=(Rw*w_4.rl-v_xw4.rl)/(abs(Rw*w_4.rl+v_xw4.rl)/2);
s_x4.rr=(Rw*w_4.rr-v_xw4.rr)/(abs(Rw*w_4.rr+v_xw4.rr)/2);

s_y4.fl=v_yw4.fl/(abs(Rw*w_4.fl+v_xw4.fl)/2);
s_y4.fr=v_yw4.fr/(abs(Rw*w_4.fr+v_xw4.fr)/2);
s_y4.rl=v_yw4.rl/(abs(Rw*w_4.rl+v_xw4.rl)/2);
s_y4.rr=v_yw4.rr/(abs(Rw*w_4.rr+v_xw4.rr)/2);

s_xy4.fl=sqrt(s_x4.fl^2+s_y4.fl^2);
s_xy4.fr=sqrt(s_x4.fr^2+s_y4.fr^2);
s_xy4.rl=sqrt(s_x4.rl^2+s_y4.rl^2);
s_xy4.rr=sqrt(s_x4.rr^2+s_y4.rr^2);

== matlab function AllPurposeModel_TyreRelaxation/Vehicle/Wheels, Tyres & Suspsension/Tyres /Tyre-Slip Force ==
  data: s_xy4 input Bus: whl_vec4; F_xywSS4 output Bus: whl_vec4; F_z4 input Bus: whl_vec4; Par parameter
function F_xywSS4  = TyreModel(s_xy4, F_z4, Par)
%#codegen

C0=Par.Veh.C0; 
mu=Par.Env.mu;
Rw=Par.Veh.Rw;

F_xywSS4.fl = min(C0*s_xy4.fl, mu) * max(F_z4.fl, 0);
F_xywSS4.fr = min(C0*s_xy4.fr, mu) * max(F_z4.fr, 0);
F_xywSS4.rl = min(C0*s_xy4.rl, mu) * max(F_z4.rl, 0);
F_xywSS4.rr = min(C0*s_xy4.rr, mu) * max(F_z4.rr, 0);


% if s_xy4.fl>Par.Env.mu/Par.Veh.C0
%     F_xywSS4.fl=min(C0*s_xy4.fl,mu)*max(F_z4.fl,0);
% else
%     F_xw4.fl=+max(F_z4.fl,0)*Par.Veh.C0*s_x4.fl;
%     F_yw4.fl=-max(F_z4.fl,0)*Par.Veh.C0*s_y4.fl;
% end

== matlab function AllPurposeModel_TyreRelaxation/Vehicle/Wheels, Tyres & Suspsension/Springs, Dampers & Linkage/Suspension Equilibrium ==
  data: T_s4 input Bus: whl_vec4; F_sd4 input Bus: whl_vec4; F_z4 output Bus: whl_vec4; F_xv4 input Bus: whl_vec4; F_yv4 input Bus: whl_vec4; delta_w4 input Bus: whl_vec4; Par parameter
function F_z4   = SuspEquil(T_s4, F_sd4, F_xv4,F_yv4,delta_w4, Par)
%#codegen

F_z4.fl = F_sd4.fl +(+T_s4.fl*(cos(delta_w4.fl)*Par.Veh.r_lever.fl(2) -Par.Veh.r_lever.fl(1)*sin(delta_w4.fl))...
    -F_xv4.fl*(Par.Veh.r_lever.fl(2)*Par.Veh.r_pivot.fl(3)+Par.Veh.r_lever.fl(3)*Par.Veh.r_pivot.fl(2)) ...
    +F_yv4.fl*(Par.Veh.r_lever.fl(1)*Par.Veh.r_pivot.fl(3)-Par.Veh.r_lever.fl(3)*Par.Veh.r_pivot.fl(1))) ...
    /(Par.Veh.r_lever.fl(1)*Par.Veh.r_pivot.fl(2)-Par.Veh.r_lever.fl(2)*Par.Veh.r_pivot.fl(1));
F_z4.fr = F_sd4.fr +(+T_s4.fr*(cos(delta_w4.fr)*Par.Veh.r_lever.fr(2) -Par.Veh.r_lever.fr(1)*sin(delta_w4.fr))...
    -F_xv4.fr*(Par.Veh.r_lever.fr(2)*Par.Veh.r_pivot.fr(3)+Par.Veh.r_lever.fr(3)*Par.Veh.r_pivot.fr(2)) ...
    +F_yv4.fr*(Par.Veh.r_lever.fr(1)*Par.Veh.r_pivot.fr(3)-Par.Veh.r_lever.fr(3)*Par.Veh.r_pivot.fr(1))) ...
    /(Par.Veh.r_lever.fr(1)*Par.Veh.r_pivot.fr(2)-Par.Veh.r_lever.fr(2)*Par.Veh.r_pivot.fr(1));
F_z4.rl = F_sd4.rl +(+T_s4.rl*(cos(delta_w4.rl)*Par.Veh.r_lever.rl(2) -Par.Veh.r_lever.rl(1)*sin(delta_w4.rl))...
    -F_xv4.rl*(Par.Veh.r_lever.rl(2)*Par.Veh.r_pivot.rl(3)+Par.Veh.r_lever.rl(3)*Par.Veh.r_pivot.rl(2)) ...
    +F_yv4.rl*(Par.Veh.r_lever.rl(1)*Par.Veh.r_pivot.rl(3)-Par.Veh.r_lever.rl(3)*Par.Veh.r_pivot.rl(1))) ...
    /(Par.Veh.r_lever.rl(1)*Par.Veh.r_pivot.rl(2)-Par.Veh.r_lever.rl(2)*Par.Veh.r_pivot.rl(1));
F_z4.rr = F_sd4.rr +(+T_s4.rr*(cos(delta_w4.rr)*Par.Veh.r_lever.rr(2) -Par.Veh.r_lever.rr(1)*sin(delta_w4.rr))...
    -F_xv4.rr*(Par.Veh.r_lever.rr(2)*Par.Veh.r_pivot.rr(3)+Par.Veh.r_lever.rr(3)*Par.Veh.r_pivot.rr(2)) ...
    +F_yv4.rr*(Par.Veh.r_lever.rr(1)*Par.Veh.r_pivot.rr(3)-Par.Veh.r_lever.rr(3)*Par.Veh.r_pivot.rr(1))) ...
    /(Par.Veh.r_lever.rr(1)*Par.Veh.r_pivot.rr(2)-Par.Veh.r_lever.rr(2)*Par.Veh.r_pivot.rr(1));

% h1f=Par.Veh.hf;
% h2f=h1f;
% h3f=Par.Veh.hf;
% h4f=h3f;
% 
% f1=Par.Veh.ff;
% f2=-f1;
% f3=Par.Veh.fr;
% f4=-f3;
% 
% F_z4.fl=(0*F_xv4.fl +h1f*F_yv4.fl +0*T_s4.fl +(-f1)*F_sd4.fl)/(-f1);
% F_z4.fr=(0*F_xv4.fr +h2f*F_yv4.fr +0*T_s4.fr +(-f2)*F_sd4.fr)/(-f2);
% F_z4.rl=(0*F_xv4.rl +h3f*F_yv4.rl +0*T_s4.rl +(-f3)*F_sd4.rl)/(-f3);
% F_z4.rr=(0*F_xv4.rr +h4f*F_yv4.rr +0*T_s4.rr +(-f4)*F_sd4.rr)/(-f4);

== matlab function AllPurposeModel_TyreRelaxation/Vehicle/Wheels, Tyres & Suspsension/Tyres /Tyre Relaxation ==
  data: w_4 input Bus: whl_vec4; F_xywSS4 input; derF_xyw4 output Bus: whl_vec4; F_xyw4 input Bus: whl_vec4; Par parameter
function derF_xyw4   = TyreModel(w_4, F_xywSS4, F_xyw4, Par)
%#codegen

derF_xyw4.fl=(F_xywSS4.fl-F_xyw4.fl)*abs(Par.Veh.Rw*w_4.fl)/Par.Veh.RelaxLength;
derF_xyw4.fr=(F_xywSS4.fr-F_xyw4.fr)*abs(Par.Veh.Rw*w_4.fr)/Par.Veh.RelaxLength;
derF_xyw4.rl=(F_xywSS4.rl-F_xyw4.rl)*abs(Par.Veh.Rw*w_4.rl)/Par.Veh.RelaxLength;
derF_xyw4.rr=(F_xywSS4.rr-F_xyw4.rr)*abs(Par.Veh.Rw*w_4.rr)/Par.Veh.RelaxLength;

== matlab function AllPurposeModel_TyreRelaxation/Vehicle/Vehicle Motion/Whole Vehicle IRP/Vehicle Velocity in-road-plane ==
  data: F_xv4 input Bus: whl_vec4; F_yv4 input Bus: whl_vec4; v_irp3 input Bus: irp_vec3; Par parameter; derv_irp3 output Bus: irp_vec3
function derv_irp3  = Body_irp(F_xv4,F_yv4, v_irp3, Par)
%old: function derv_irp3  = Body_irp(F_1xv,F_2xv,F_3xv,F_4xv, F_1yv,F_2yv,F_3yv,F_4yv, v_irp3, Par)
%#codegen

v_x=v_irp3.x;
v_y=v_irp3.y;
w_z=v_irp3.rotz;

lf=Par.Veh.lf;
lr=Par.Veh.lr;

w1=Par.Veh.TrackWidth/2;
w2=-w1;
w3=w1;
w4=-w3;

T_irpv=[[ 1   1   1   1 ] [0  0  0  0 ]; ...
    [ 0   0   0   0 ] [1  1  1  1 ]; ...
    [-w1 -w2 -w3 -w4] [lf lf lr lr]];

F_xv4_temp=[F_xv4.fl;F_xv4.fr;F_xv4.rl;F_xv4.rr];
F_yv4_temp=[F_yv4.fl;F_yv4.fr;F_yv4.rl;F_yv4.rr];

F_air=Par.Veh.HalfRohACd*abs(v_x)*v_x;
beta=atan2(v_y,v_x);

derv_irp3_temp=diag([1/Par.Veh.m 1/Par.Veh.m 1/Par.Veh.Jz])*(T_irpv*[F_xv4_temp;F_yv4_temp]-[sin(beta);sin(beta);0]*F_air)-[-v_y*w_z; +v_x*w_z; 0];

derv_irp3 = struct('x',derv_irp3_temp(1),'y',derv_irp3_temp(2),'rotz',derv_irp3_temp(3));

== matlab function AllPurposeModel_TyreRelaxation/Vehicle/Vehicle Motion/Whole Vehicle IRP/Vehicle Position in-road-plane ==
  data: v_irp3 input Bus: irp_vec3; p_z input; derpos_irp3 output Bus: irp_vec3
function derpos_irp3  = BodyPath_irp(v_irp3, p_z)
%#codegen

derpos_irp3.x   = cos(p_z)*v_irp3.x -sin(p_z)*v_irp3.y;
derpos_irp3.y   = sin(p_z)*v_irp3.x +cos(p_z)*v_irp3.y;
derpos_irp3.rotz= v_irp3.rotz;

== matlab function AllPurposeModel_TyreRelaxation/Vehicle/Wheels, Tyres & Suspsension/Springs, Dampers & Linkage/Dampers ==
  data: v_z4 input Bus: whl_vec4; F_d4 output Bus: whl_vec4; Par parameter
function F_d4   =  Dampers(v_z4,Par)
%old: function [F_1d,F_2d,F_3d,F_4d]  =  Dampers(v_1z,v_2z,v_3z,v_4z,Par)
%#codegen

d1=Par.Veh.dw;
d2=Par.Veh.dw;
d3=Par.Veh.dw;
d4=Par.Veh.dw;

F_d4.fl=-d1*v_z4.fl;
F_d4.fr=-d2*v_z4.fr;
F_d4.rl=-d3*v_z4.rl;
F_d4.rr=-d4*v_z4.rr;

== matlab function AllPurposeModel_TyreRelaxation/Vehicle/Wheels, Tyres & Suspsension/Springs, Dampers & Linkage/Springs ==
  data: v_z4 input Bus: whl_vec4; derF_s4 output Bus: whl_vec4; Par parameter
function derF_s4   = Springs(v_z4,Par)
%old: function [derF_1s,derF_2s,derF_3s,derF_4s]  = Springs(v_1z,v_2z,v_3z,v_4z,Par)
%#codegen

derF_s4.fl=[Par.Veh.cw, Par.Veh.carb_f]*[-v_z4.fl; -v_z4.fr];
derF_s4.fr=[Par.Veh.cw, Par.Veh.carb_f]*[-v_z4.fr; -v_z4.fl];
derF_s4.rl=[Par.Veh.cw, Par.Veh.carb_r]*[-v_z4.rl; -v_z4.rr];
derF_s4.rr=[Par.Veh.cw, Par.Veh.carb_r]*[-v_z4.rr; -v_z4.rl];

== matlab function AllPurposeModel_TyreRelaxation/Vehicle/Vehicle Motion/Sprung Body OORP/Body OORP ==
  data: F_xv4 input Bus: whl_vec4; derv_oorp3 output Bus: oorp_vec3; F_yv4 input Bus: whl_vec4; F_z4 input Bus: whl_vec4; Par parameter
function derv_oorp3   = fcn(F_xv4,F_yv4, F_z4, Par)
%old: function derv_oorp3   = fcn(F_1xv,F_2xv,F_3xv,F_4xv, F_1yv,F_2yv,F_3yv,F_4yv, F_1z,F_2z,F_3z,F_4z, Par)
%#codegen

w1=Par.Veh.TrackWidth/2; %"half wheel base" #Can notation w1 conflict with wheel rotational speed?
w2=-w1;
w3=w1;
w4=w2;

lf=Par.Veh.lf;
lr=Par.Veh.lr;

h=Par.Veh.h; 

T_oorpv=[[ 1   1   1   1 ];...
         [ w1  w2  w3  w4];...
         [-lf -lf -lr -lr]];

F_xv4_temp=[F_xv4.fl;F_xv4.fr;F_xv4.rl;F_xv4.rr];
F_yv4_temp=[F_yv4.fl;F_yv4.fr;F_yv4.rl;F_yv4.rr];
F_z4_temp =[F_z4.fl; F_z4.fr; F_z4.rl; F_z4.rr];

     
F_oorp3=...
[[0 0 0 0; 0 0 0 0; -h -h -h -h]*F_xv4_temp+...
 [0 0 0 0; h h h h;  0  0  0  0]*F_yv4_temp+...
 T_oorpv*F_z4_temp]+[-Par.Veh.m*Par.Env.g;0;0];

derv_oorp3.z=F_oorp3(1)/Par.Veh.m_sprung;
derv_oorp3.rotx=F_oorp3(2)/Par.Veh.Jx_sprung;
derv_oorp3.roty=F_oorp3(3)/Par.Veh.Jy_sprung;

== matlab function AllPurposeModel_TyreRelaxation/Vehicle/Vehicle Motion/Compatibility IRP/Compatibility ==
  data: v_xv4 output Bus: whl_vec4; v_yv4 output Bus: whl_vec4; v_irp3 input Bus: irp_vec3; Par parameter
function [v_xv4,v_yv4] = fcn(v_irp3,Par)
%old: function [v_1xv,v_2xv,v_3xv,v_4xv, v_1yv,v_2yv,v_3yv,v_4yv] = fcn(v_x,v_y,w_z,Par)
%#codegen

lf=Par.Veh.lf;
lr=Par.Veh.lr;

w1=Par.Veh.TrackWidth/2;
w2=-w1;
w3=w1;
w4=-w3;

T_irpv=[[ 1   1   1   1 ] [0  0  0  0 ]; ...
        [ 0   0   0   0 ] [1  1  1  1 ]; ...
        [-w1 -w2 -w3 -w4] [lf lf lr lr]];

v_irp3_temp=[v_irp3.x; v_irp3.y; v_irp3.rotz];
 
v_xyv8=T_irpv'*v_irp3_temp;

v_xv4=struct('fl',v_xyv8(1),'fr',v_xyv8(2),'rl',v_xyv8(3),'rr',v_xyv8(4));
v_yv4=struct('fl',v_xyv8(5),'fr',v_xyv8(6),'rl',v_xyv8(7),'rr',v_xyv8(8));
